simulink model "quadcopter_2016a_0211"  (R2016a)
settings: Solver=ode45  SolverMode=SingleTasking  StartTime=0.0  StopTime=30  RelTol=1e-3
values from neighbouring files (symbols this model uses):
  b = 5.9347e-06    [parameters.m]
  d = 1.2181e-07    [parameters.m]
  g = 9.81    [parameters.m]
  I = diag([Ix,Iy,Iz])    [parameters.m]
  Ix = 0.0073    [parameters.m]
  Iy = 0.0073    [parameters.m]
  Iz = 0.0117    [parameters.m]
  Kd = d*lambda    [parameters.m]
  ks = 735    [parameters.m]
  Kth = b*lambda    [parameters.m]
  L = 0.17    [parameters.m]
  m = 0.616    [parameters.m]
  tau = 1/200    (= 0.005)    [parameters.m]
  u0 = 0.49    [parameters.m]
undefined symbols (not defined in the file or in its folder): attitudeinit, Kp1_pitch, Kp1_roll, Kp1_yaw, Kp2_pitch, Kp2_roll, Kp2_yaw, kxir, kxir_th, omegainit, posinit, velinit, wr_n, wr_n_th
settings Model: Creator=LENOVO  LastModifiedBy=ASUS
settings SolverCC: ZeroCrossAlgorithm=Adaptive
settings DataIOCC: ReturnWorkspaceOutputs=on  Refine=2
settings DebuggingCC: MaskedZcDiagnostic=none  IgnoredZcDiagnostic=none  SFUnexpectedBacktrackingDiag=error  SFNoUnconditionalDefaultTransitionDiag=error
settings SFSimCC: SimUseLocalCustomCode=on
settings RTWCC: RTWUseLocalCustomCode=on
settings GRTTargetCC: TargetLangStandard=C99 (ISO)  GeneratePreprocessorConditionals=Use local settings
settings ConfigComp: CovMetricSettings=dwe  CovSaveCumulativeToWorkspaceVar=off  CovSaveSingleToWorkspaceVar=off  CovExternalEMLEnable=on

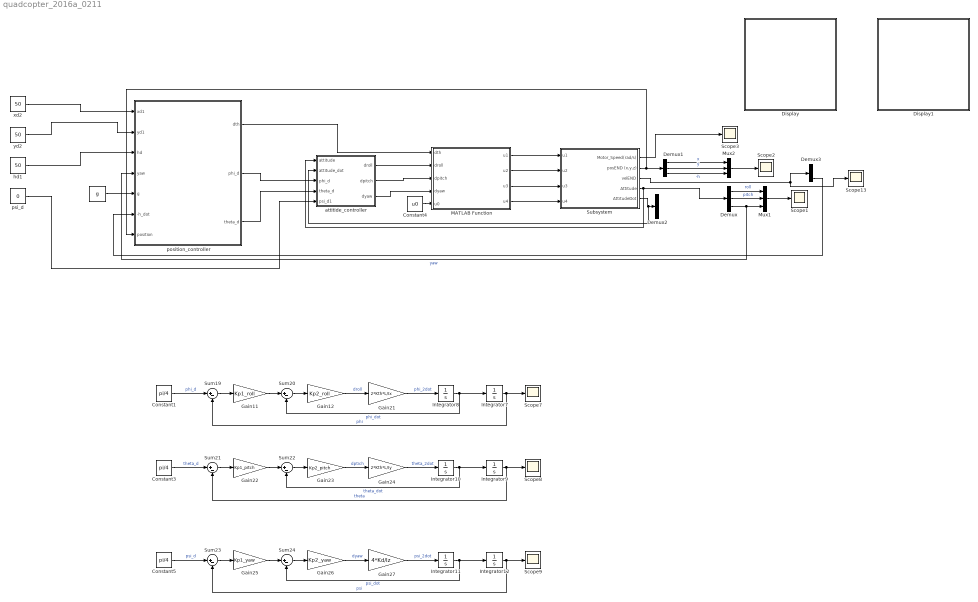
== system quadcopter_2016a_0211 ==
  " " : Constant  Value=g
  Constant1 : Constant  Value=pi/4
  Constant3 : Constant  Value=pi/4
  Constant4 : Constant  Value=u0
  Constant5 : Constant  Value=pi/4
  Demux{,1..3} (4 alike) : Demux  Outputs=3
  Display : Subsystem  Description=Replaced Block  mask(Replaced Block){}
      mask help: This block has been replaced with an empty subsystem because it used functionality that is unavailable in Simulink R2016a.
      mask Display: fprintf('Replaced: %s\n','Dashboard Widget')
  Display1 : Subsystem  Description=Replaced Block  mask(Replaced Block){}
      mask help: This block has been replaced with an empty subsystem because it used functionality that is unavailable in Simulink R2016a.
      mask Display: fprintf('Replaced: %s\n','Dashboard Widget')
  Gain11 : Gain  Gain=Kp1_roll
  Gain12 : Gain  Gain=Kp2_roll
  Gain21 : Gain  Gain=2*Kth*L/Ix
  Gain22 : Gain  Gain=Kp1_pitch
  Gain23 : Gain  Gain=Kp2_pitch
  Gain24 : Gain  Gain=2*Kth*L/Iy
  Gain25 : Gain  Gain=Kp1_yaw
  Gain26 : Gain  Gain=Kp2_yaw
  Gain27 : Gain  Gain=4*Kd/Iz
  Integrator{7..12} (6 alike) : Integrator
  MATLAB Function : MATLAB Function  TreatAsAtomicUnit=on
  Mux1 : Mux  Inputs=3
  Mux2 : Mux  Inputs=3
  Scope{1..3,7..9,13} (7 alike) : Scope
  Subsystem : Subsystem
  Sum{19..24} (6 alike) : Sum  Inputs=|+-
  attitide_controller : Subsystem
  hd1 : Constant  Value=50
  position_controller : Subsystem
  psi_d : Constant  Value=0
  xd2 : Constant  Value=50
  yd2 : Constant  Value=50
  wires:
  MATLAB Function/2(u2) -> Subsystem/2(u2)
  Demux1/1 -> Mux2/1  "x"
  Subsystem/2(posEND (x,y,z)) -> position_controller/7(position), Demux1/1
  Demux1/2 -> Mux2/2  "y"
  Mux1/1 -> Scope1/1
  MATLAB Function/1(u1) -> Subsystem/1(u1)
  Constant4/1 -> MATLAB Function/5(u0)
  Demux/2 -> Mux1/2  "pitch"
  Subsystem/5(AttitudeDot) -> attitide_controller/2(attitude_dot), Demux2/1
  MATLAB Function/3(u3) -> Subsystem/3(u3)
  MATLAB Function/4(u4) -> Subsystem/4(u4)
  Subsystem/4(Attitude) -> Demux/1, attitide_controller/1(attitude)
  Demux/1 -> Mux1/1  "roll"
  Mux2/1 -> Scope2/1
  Demux/3 -> position_controller/4(yaw), Mux1/3  "yaw"
  Gain11/1 -> Sum20/1
  Sum20/1 -> Gain12/1
  Constant1/1 -> Sum19/1  "phi_d"
  Gain12/1 -> Gain21/1  "droll"
  Sum19/1 -> Gain11/1
  Integrator7/1 -> Scope7/1, Sum19/2  "phi"
  Gain21/1 -> Integrator8/1  "phi_2dot"
  Integrator8/1 -> Integrator7/1, Sum20/2  "phi_dot"
  Gain24/1 -> Integrator10/1  "theta_2dot"
  Integrator10/1 -> Integrator9/1, Sum22/2  "theta_dot"
  Gain22/1 -> Sum22/1
  Integrator9/1 -> Scope8/1, Sum21/2  "theta"
  Sum22/1 -> Gain23/1
  Gain23/1 -> Gain24/1  "dptich"
  Constant3/1 -> Sum21/1  "theta_d"
  Sum21/1 -> Gain22/1
  Sum23/1 -> Gain25/1
  Gain26/1 -> Gain27/1  "dyaw"
  Integrator12/1 -> Scope9/1, Sum23/2  "psi"
  Gain25/1 -> Sum24/1
  Integrator11/1 -> Integrator12/1, Sum24/2  "psi_dot"
  Sum24/1 -> Gain26/1
  Constant5/1 -> Sum23/1  "psi_d"
  Gain27/1 -> Integrator11/1  "psi_2dot"
  Subsystem/3(velEND) -> Demux3/1, Scope13/1
  Demux1/3 -> Mux2/3  "-h"
  psi_d/1 -> attitide_controller/5(psi_d1)
  attitide_controller/1(droll) -> MATLAB Function/2(droll)
  attitide_controller/2(dpitch) -> MATLAB Function/3(dpitch)
  attitide_controller/3(dyaw) -> MATLAB Function/4(dyaw)
  " "/1 -> position_controller/5(g)
  yd2/1 -> position_controller/2(yd1)
  hd1/1 -> position_controller/3(hd)
  xd2/1 -> position_controller/1(xd1)
  position_controller/2(phi_d) -> attitide_controller/3(phi_d)
  position_controller/3(theta_d) -> attitide_controller/4(theta_d)
  position_controller/1(dth) -> MATLAB Function/1(dth)
  Demux3/3 -> position_controller/6(-h_dot)
  Subsystem/1(Motor_Speed(rad/s)) -> Scope3/1

== system quadcopter_2016a_0211/Display ==

== system quadcopter_2016a_0211/Display1 ==

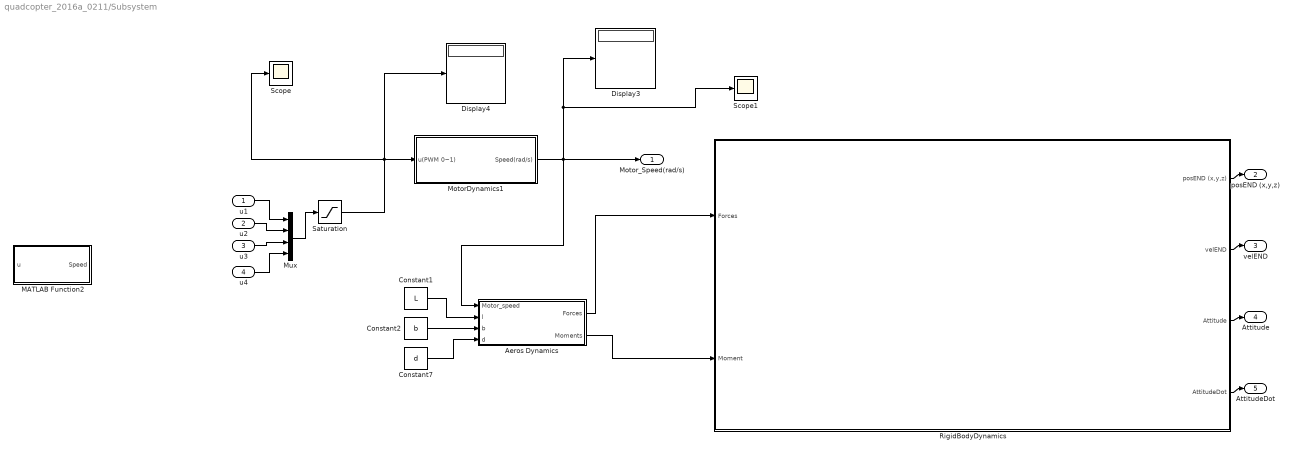
== system quadcopter_2016a_0211/Subsystem ==
  u1 : Inport  Description=u1
  u2 : Inport  Port=2
  u3 : Inport  Port=3
  u4 : Inport  Port=4
  Aeros Dynamics : MATLAB Function  TreatAsAtomicUnit=on
  Constant1 : Constant  Value=L
  Constant2 : Constant  Value=b
  Constant7 : Constant  Value=d
  Display3 : Display
  Display4 : Display
  MATLAB Function2 : MATLAB Function  TreatAsAtomicUnit=on
  MotorDynamics1 : Subsystem
  Mux : Mux
  RigidBodyDynamics : Subsystem
  Saturation : Saturate  UpperLimit=1  LowerLimit=0
  Scope : Scope
  Scope1 : Scope
  Motor_Speed(rad/s) : Outport
  posEND (x,y,z) : Outport  Port=2
  velEND : Outport  Port=3
  Attitude : Outport  Port=4
  AttitudeDot : Outport  Port=5
  wires:
  Constant1/1 -> Aeros Dynamics/2(l)
  u2/1 -> Mux/2
  u4/1 -> Mux/4
  u1/1 -> Mux/1
  Constant7/1 -> Aeros Dynamics/4(d)
  Aeros Dynamics/2(Moments) -> RigidBodyDynamics/2(Moment)
  Aeros Dynamics/1(Forces) -> RigidBodyDynamics/1(Forces)
  Constant2/1 -> Aeros Dynamics/3(b)
  MotorDynamics1/1(Speed(rad/s)) -> Aeros Dynamics/1(Motor_speed), Scope1/1, Display3/1, Motor_Speed(rad/s)/1
  u3/1 -> Mux/3
  RigidBodyDynamics/4(AttitudeDot) -> AttitudeDot/1
  RigidBodyDynamics/3(Attitude) -> Attitude/1
  RigidBodyDynamics/2(velEND) -> velEND/1
  RigidBodyDynamics/1(posEND (x,y,z)) -> posEND (x,y,z)/1
  Saturation/1 -> MotorDynamics1/1(u(PWM 0~1)), Scope/1, Display4/1
  Mux/1 -> Saturation/1

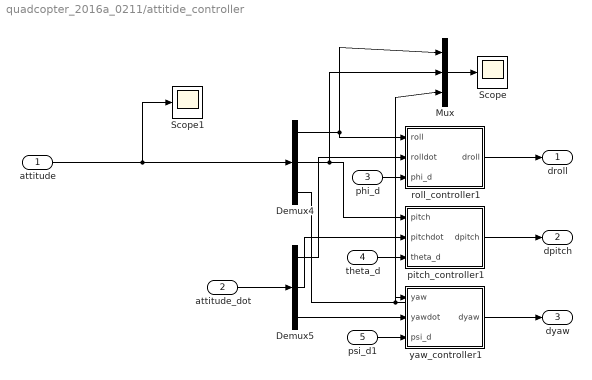
== system quadcopter_2016a_0211/attitide_controller ==
  attitude : Inport
  attitude_dot : Inport  Port=2
  phi_d : Inport  Port=3
  theta_d : Inport  Port=4
  psi_d1 : Inport  Port=5
  Demux4 : Demux  Outputs=3
  Demux5 : Demux  Outputs=3
  Mux : Mux  Inputs=3
  Scope : Scope
  Scope1 : Scope
  pitch_controller1 : Subsystem
  roll_controller1 : Subsystem
  yaw_controller1 : Subsystem
  droll : Outport
  dpitch : Outport  Port=2
  dyaw : Outport  Port=3
  wires:
  attitude_dot/1 -> Demux5/1
  yaw_controller1/1(dyaw) -> dyaw/1
  attitude/1 -> Scope1/1, Demux4/1
  Demux5/3 -> yaw_controller1/2(yawdot)
  Demux4/3 -> Mux/3, yaw_controller1/1(yaw)
  roll_controller1/1(droll) -> droll/1
  theta_d/1 -> pitch_controller1/3(theta_d)
  Demux5/1 -> roll_controller1/2(rolldot)
  pitch_controller1/1(dpitch) -> dpitch/1
  psi_d1/1 -> yaw_controller1/3(psi_d)
  phi_d/1 -> roll_controller1/3(phi_d)
  Demux4/1 -> Mux/1, roll_controller1/1(roll)
  Demux5/2 -> pitch_controller1/2(pitchdot)
  Demux4/2 -> Mux/2, pitch_controller1/1(pitch)
  Mux/1 -> Scope/1

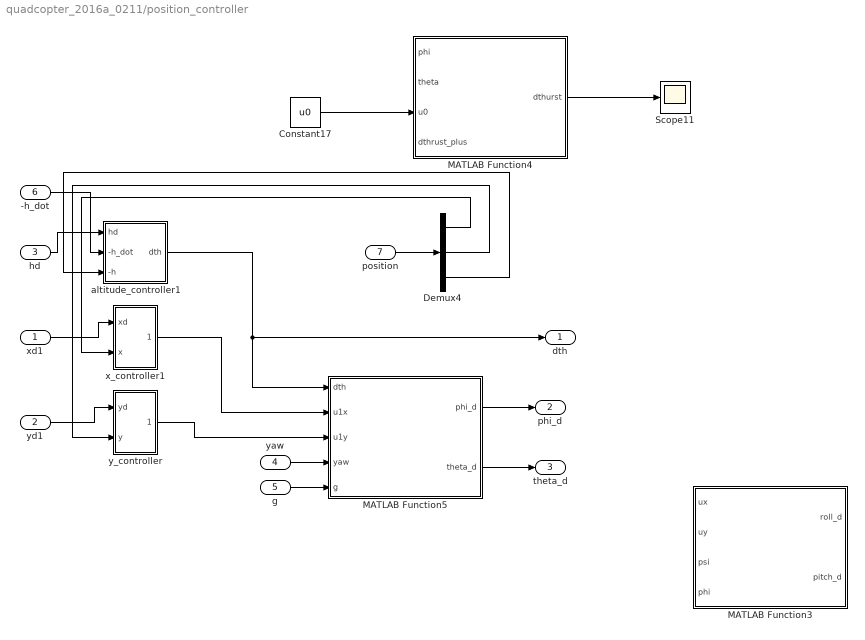
== system quadcopter_2016a_0211/position_controller ==
  xd1 : Inport
  yd1 : Inport  Port=2
  hd : Inport  Port=3
  yaw : Inport  Port=4
  g : Inport  Port=5
  -h_dot : Inport  Port=6
  position : Inport  Port=7
  Constant17 : Constant  Value=u0
  Demux4 : Demux  Outputs=3
  MATLAB Function3 : MATLAB Function  TreatAsAtomicUnit=on
  MATLAB Function4 : MATLAB Function  TreatAsAtomicUnit=on
  MATLAB Function5 : MATLAB Function  TreatAsAtomicUnit=on
  Scope11 : Scope
  altitude_controller1 : Subsystem
  x_controller1 : Subsystem
  y_controller : Subsystem
  dth : Outport
  phi_d : Outport  Port=2
  theta_d : Outport  Port=3
  wires:
  x_controller1/1(u1x) -> MATLAB Function5/2(u1x)
  Demux4/1 -> x_controller1/2(x)
  altitude_controller1/1(dth) -> dth/1, MATLAB Function5/1(dth)
  -h_dot/1 -> altitude_controller1/2(-h_dot)
  yaw/1 -> MATLAB Function5/4(yaw)
  xd1/1 -> x_controller1/1(xd)
  position/1 -> Demux4/1
  MATLAB Function5/2(theta_d) -> theta_d/1
  MATLAB Function5/1(phi_d) -> phi_d/1
  Demux4/2 -> y_controller/2(y)
  hd/1 -> altitude_controller1/1(hd)
  Demux4/3 -> altitude_controller1/3(-h)
  yd1/1 -> y_controller/1(yd)
  y_controller/1(u1y) -> MATLAB Function5/3(u1y)
  g/1 -> MATLAB Function5/5(g)
  MATLAB Function4/1(dthurst) -> Scope11/1
  Constant17/1 -> MATLAB Function4/3(u0)

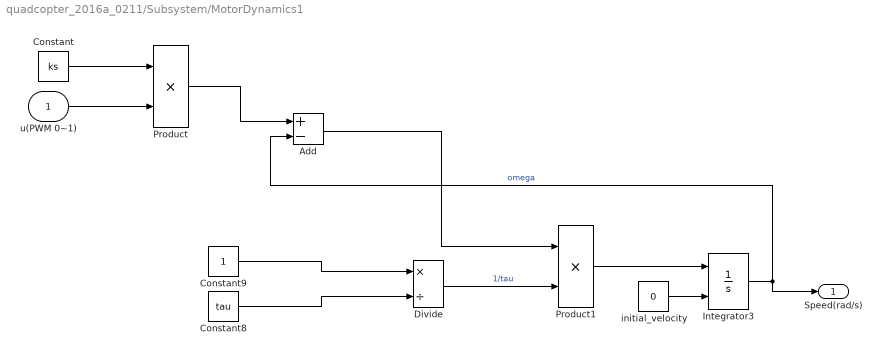
== system quadcopter_2016a_0211/Subsystem/MotorDynamics1 ==
  u(PWM 0~1) : Inport
  Add : Sum  Inputs=+-
  Constant : Constant  Value=ks
  Constant8 : Constant  Value=tau
  Constant9 : Constant
  Divide : Product  Inputs=*/
  Integrator3 : Integrator  InitialConditionSource=external  InitialCondition=omegainit
  Product : Product
  Product1 : Product
  initial_velocity : Constant  Value=0
  Speed(rad/s) : Outport
  wires:
  u(PWM 0~1)/1 -> Product/2
  Constant/1 -> Product/1
  Constant9/1 -> Divide/1
  Product1/1 -> Integrator3/1
  Constant8/1 -> Divide/2
  Divide/1 -> Product1/2  "1/tau"
  Integrator3/1 -> Add/2, Speed(rad/s)/1  "omega"
  Product/1 -> Add/1
  Add/1 -> Product1/1
  initial_velocity/1 -> Integrator3/2

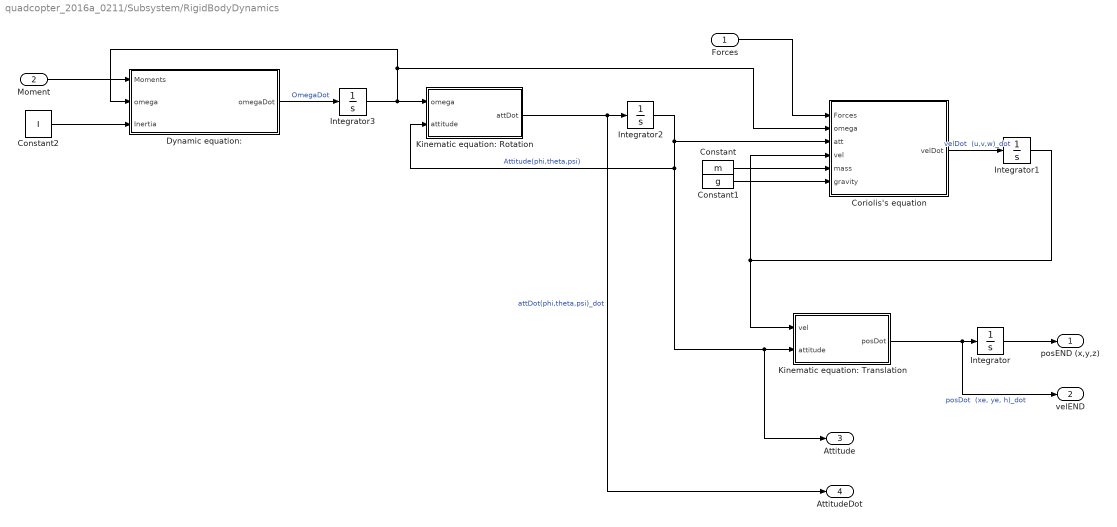
== system quadcopter_2016a_0211/Subsystem/RigidBodyDynamics ==
  Forces : Inport
  Moment : Inport  Port=2
  Constant : Constant  Value=m
  Constant1 : Constant  Value=g
  Constant2 : Constant  Value=I
  Coriolis's equation : MATLAB Function  TreatAsAtomicUnit=on
  "Dynamic equation: " : MATLAB Function  TreatAsAtomicUnit=on
  Integrator : Integrator  InitialCondition=posinit
  Integrator1 : Integrator  InitialCondition=velinit
  Integrator2 : Integrator  InitialCondition=attitudeinit
  Integrator3 : Integrator  InitialCondition=omegainit
  Kinematic equation: Rotation : MATLAB Function  TreatAsAtomicUnit=on
  Kinematic equation: Translation : MATLAB Function  TreatAsAtomicUnit=on
  posEND (x,y,z) : Outport
  velEND : Outport  Port=2
  Attitude : Outport  Port=3
  AttitudeDot : Outport  Port=4
  wires:
  Integrator2/1 -> Attitude/1, Kinematic equation: Translation/2(attitude), Kinematic equation: Rotation/2(attitude), Coriolis's equation/3(att)  "Attitude(phi,theta,psi)"
  Constant2/1 -> "Dynamic equation: "/3(Inertia)
  Coriolis's equation/1(velDot) -> Integrator1/1  "velDot  (u,v,w)_dot"
  Kinematic equation: Translation/1(posDot) -> velEND/1, Integrator/1  "posDot  (xe, ye, h)_dot"
  Constant1/1 -> Coriolis's equation/6(gravity)
  Forces/1 -> Coriolis's equation/1(Forces)
  Integrator/1 -> posEND (x,y,z)/1
  Integrator3/1 -> Kinematic equation: Rotation/1(omega), "Dynamic equation: "/2(omega), Coriolis's equation/2(omega)
  Integrator1/1 -> Kinematic equation: Translation/1(vel), Coriolis's equation/4(vel)
  Kinematic equation: Rotation/1(attDot) -> AttitudeDot/1, Integrator2/1  "attDot(phi,theta,psi)_dot"
  Moment/1 -> "Dynamic equation: "/1(Moments)
  "Dynamic equation: "/1(omegaDot) -> Integrator3/1  "OmegaDot"
  Constant/1 -> Coriolis's equation/5(mass)

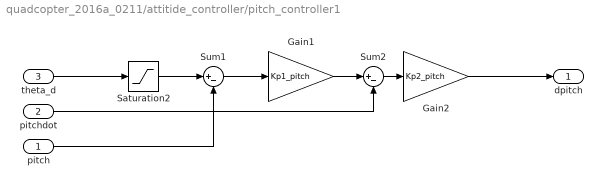
== system quadcopter_2016a_0211/attitide_controller/pitch_controller1 ==
  pitch : Inport
  pitchdot : Inport  Port=2
  theta_d : Inport  Port=3
  Gain1 : Gain  Gain=Kp1_pitch
  Gain2 : Gain  Gain=Kp2_pitch
  Saturation2 : Saturate  UpperLimit=pi/8  LowerLimit=-pi/8
  Sum1 : Sum  Inputs=|+-
  Sum2 : Sum  Inputs=|+-
  dpitch : Outport
  wires:
  Gain1/1 -> Sum2/1
  Gain2/1 -> dpitch/1
  pitch/1 -> Sum1/2
  Saturation2/1 -> Sum1/1
  Sum2/1 -> Gain2/1
  Sum1/1 -> Gain1/1
  pitchdot/1 -> Sum2/2
  theta_d/1 -> Saturation2/1

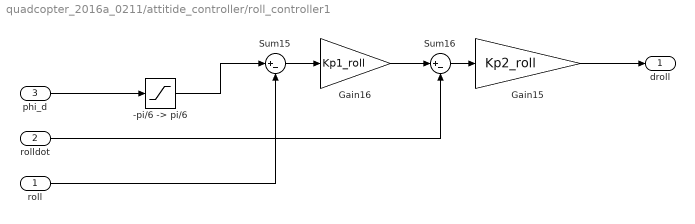
== system quadcopter_2016a_0211/attitide_controller/roll_controller1 ==
  roll : Inport
  rolldot : Inport  Port=2
  phi_d : Inport  Port=3
  "-pi/6 -> pi/6" : Saturate  UpperLimit=pi/8  LowerLimit=-pi/8
  Gain15 : Gain  Gain=Kp2_roll
  Gain16 : Gain  Gain=Kp1_roll
  Sum15 : Sum  Inputs=|+-
  Sum16 : Sum  Inputs=|+-
  droll : Outport
  wires:
  phi_d/1 -> "-pi/6 -> pi/6"/1
  rolldot/1 -> Sum16/2
  Sum16/1 -> Gain15/1
  roll/1 -> Sum15/2
  Sum15/1 -> Gain16/1
  "-pi/6 -> pi/6"/1 -> Sum15/1
  Gain15/1 -> droll/1
  Gain16/1 -> Sum16/1

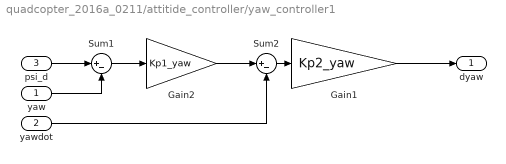
== system quadcopter_2016a_0211/attitide_controller/yaw_controller1 ==
  yaw : Inport
  yawdot : Inport  Port=2
  psi_d : Inport  Port=3
  Gain1 : Gain  Gain=Kp2_yaw
  Gain2 : Gain  Gain=Kp1_yaw
  Sum1 : Sum  Inputs=|+-
  Sum2 : Sum  Inputs=|+-
  dyaw : Outport
  wires:
  psi_d/1 -> Sum1/1
  Sum2/1 -> Gain1/1
  Gain2/1 -> Sum2/1
  yaw/1 -> Sum1/2
  Sum1/1 -> Gain2/1
  yawdot/1 -> Sum2/2
  Gain1/1 -> dyaw/1

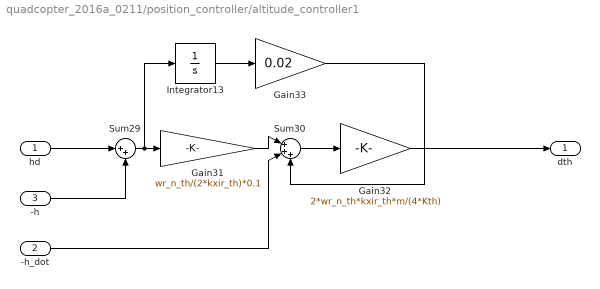
== system quadcopter_2016a_0211/position_controller/altitude_controller1 ==
  hd : Inport  Description=hd
  -h_dot : Inport  Description=hd  Port=2
  -h : Inport  Description=hd  Port=3
  Gain31 : Gain  Gain=wr_n_th/(2*kxir_th)*0.1
  Gain32 : Gain  Gain=2*wr_n_th*kxir_th*m/(4*Kth)
  Gain33 : Gain  Gain=0.02
  Integrator13 : Integrator
  Sum29 : Sum  Inputs=|++
  Sum30 : Sum  Inputs=|+++
  dth : Outport
  wires:
  -h_dot/1 -> Sum30/2
  Sum30/1 -> Gain32/1
  Integrator13/1 -> Gain33/1
  Sum29/1 -> Integrator13/1, Gain31/1
  hd/1 -> Sum29/1
  -h/1 -> Sum29/2
  Gain33/1 -> Sum30/3
  Gain31/1 -> Sum30/1
  Gain32/1 -> dth/1

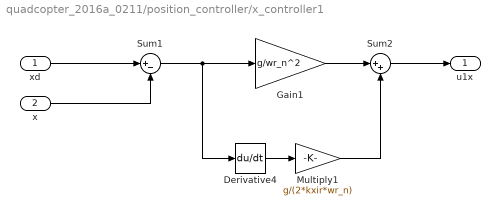
== system quadcopter_2016a_0211/position_controller/x_controller1 ==
  xd : Inport
  x : Inport  Port=2
  Derivative4 : Derivative
  Gain1 : Gain  Gain=g/wr_n^2
  Multiply1 : Gain  Gain=g/(2*kxir*wr_n)
  Sum1 : Sum  Inputs=|+-
  Sum2 : Sum  Inputs=|++
  u1x : Outport
  wires:
  Multiply1/1 -> Sum2/2
  Derivative4/1 -> Multiply1/1
  Gain1/1 -> Sum2/1
  x/1 -> Sum1/2
  xd/1 -> Sum1/1
  Sum1/1 -> Derivative4/1, Gain1/1
  Sum2/1 -> u1x/1

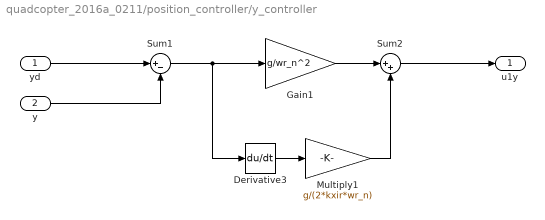
== system quadcopter_2016a_0211/position_controller/y_controller ==
  yd : Inport
  y : Inport  Port=2
  Derivative3 : Derivative
  Gain1 : Gain  Gain=g/wr_n^2
  Multiply1 : Gain  Gain=g/(2*kxir*wr_n)
  Sum1 : Sum  Inputs=|+-
  Sum2 : Sum  Inputs=|++
  u1y : Outport
  wires:
  Sum2/1 -> u1y/1
  Sum1/1 -> Derivative3/1, Gain1/1
  Gain1/1 -> Sum2/1
  Multiply1/1 -> Sum2/2
  yd/1 -> Sum1/1
  Derivative3/1 -> Multiply1/1
  y/1 -> Sum1/2

== matlab function quadcopter_2016a_0211/Subsystem/RigidBodyDynamics/Kinematic equation: Rotation ==
  data: omega input; attDot output; attitude input
function attDot = fcn(omega, attitude)
phi = attitude(1);
theta = attitude(2);
psi = attitude(3);

R = [1 sin(phi)*tan(theta) cos(phi)*tan(theta); 0 cos(phi) -sin(phi); 0 sin(phi)/cos(theta) cos(phi)/cos(theta)];

attDot = R*omega;

== matlab function quadcopter_2016a_0211/Subsystem/RigidBodyDynamics/Kinematic equation: Translation ==
  data: vel input; posDot output; attitude input
function posDot = fcn(vel, attitude)
phi = attitude(1);
theta = attitude(2);
psi = attitude(3);

R = [cos(psi)*cos(theta) cos(psi)*sin(phi)*sin(theta)-cos(phi)*sin(psi) sin(psi)*sin(phi)+cos(psi)*cos(phi)*sin(theta);
    sin(psi)*cos(theta) cos(psi)*cos(phi)+sin(psi)*sin(phi)*sin(theta) cos(phi)*sin(psi)*sin(theta)-cos(psi)*sin(phi);
    -sin(theta) cos(theta)*sin(phi) cos(phi)*cos(theta)];
% Velocity output x_dot, y_dot, z_dot [E]
posDot = R*vel;

== matlab function quadcopter_2016a_0211/Subsystem/RigidBodyDynamics/Coriolis's equation ==
  data: Forces input; omega input; att input; vel input; velDot output; mass input; gravity input
function velDot = fcn(Forces, omega, att, vel, mass, gravity)
phi = att(1);
theta = att(2);
psi = att(3);

G = [-sin(theta); sin(phi)*cos(theta); cos(phi)*cos(theta)]*gravity;

velDot = G + 1/mass * Forces - cross(omega, vel);

== matlab function quadcopter_2016a_0211/Subsystem/RigidBodyDynamics/Dynamic equation:  ==
  data: Moments input; omegaDot output; omega input; Inertia input
function omegaDot = fcn(Moments, omega, Inertia)
omegaDot = Inertia^(-1)*(Moments-cross(omega, Inertia*omega));

== matlab function quadcopter_2016a_0211/Subsystem/Aeros Dynamics ==
  data: Motor_speed input; Forces output; Moments output; l input; b input; d input
function [Forces, Moments] = fcn(Motor_speed, l, b, d)
omega1 = Motor_speed(1);
omega2 = Motor_speed(2);
omega3 = Motor_speed(3);
omega4 = Motor_speed(4);
F = b*(omega1^2 + omega2^2 + omega3^2 + omega4^2);
Forces = [0;0;-F];
Tau_x = l*b*(omega4^2-omega2^2);
Tau_y = l*b*(omega1^2-omega3^2);
Tau_z = d*(-omega1^2 + omega2^2 - omega3^2 + omega4^2);
Moments = [Tau_x; Tau_y; Tau_z];

== matlab function quadcopter_2016a_0211/MATLAB Function ==
  data: dth input; u1 output; droll input; dpitch input; dyaw input; u0 input; u2 output; u3 output; u4 output
function [u1, u2, u3, u4] = fcn(dth, droll, dpitch, dyaw, u0)
U = [ 0 1 -1; 1 -1 0 1; 1 0 -1 -1; 1 1 0 1]*[dth+u0; droll; dpitch; dyaw];
u1 = U(1);
u2 = U(2);
u3 = U(3);
u4 = U(4);1

== matlab function quadcopter_2016a_0211/Subsystem/MATLAB Function2 ==
  data: u input; Speed output
function Speed = fcn(u)
    Speed = u.*735/(1+1/2000);

== matlab function quadcopter_2016a_0211/position_controller/MATLAB Function3 ==
  data: ux input; uy input; roll_d output; psi input; pitch_d output; phi input
function [roll_d, pitch_d] = fcn(ux,uy,psi, phi)
ux = -ux;
uy = -uy;
sin_roll_d = ux*sin(psi) - uy*cos(psi);
sin_pitch_d = (ux*cos(psi)+uy*sin(psi))/cos(phi);
sin_roll_d = max(min(sin_roll_d,1),-1);
sin_pitch_d = max(min(sin_pitch_d,1),-1);
roll_d = asin(sin_roll_d);
pitch_d = asin(sin_pitch_d);

== matlab function quadcopter_2016a_0211/position_controller/MATLAB Function4 ==
  data: phi input; theta input; dthurst output; u0 input; dthrust_plus input
function dthurst = fcn(phi, theta, u0,dthrust_plus)

dthurst = (u0+dthrust_plus)/(cos(phi)*cos(theta)) - u0;

== matlab function quadcopter_2016a_0211/position_controller/MATLAB Function5 ==
  data: dth input; u1x input; phi_d output; u1y input; yaw input; g input; theta_d output
function [phi_d, theta_d] = fcn(dth, u1x, u1y, yaw, g)
u1z=dth+g;
u1x=-u1x;
u1y = -u1y;
phi_d = atan2(sin(yaw)*cos(yaw)*u1x-cos(yaw)^2*u1y, u1z);
sin_theta_d = cos(yaw)^2*u1x+sin(yaw)*cos(yaw)*u1y/ u1z;
sin_theta_d = max(min(sin_theta_d, 1), -1);
theta_d = asin(sin_theta_d);
